simulink library "libaeolus_at"  (Simulink 7.9)
settings: Solver=ode45  StartTime=0.0  StopTime=10.0  RelTol=1e-3
undefined symbols (not defined in the file or in its folder): sigbuilder_block
libraries: simulink x3
(part 2 of 2)

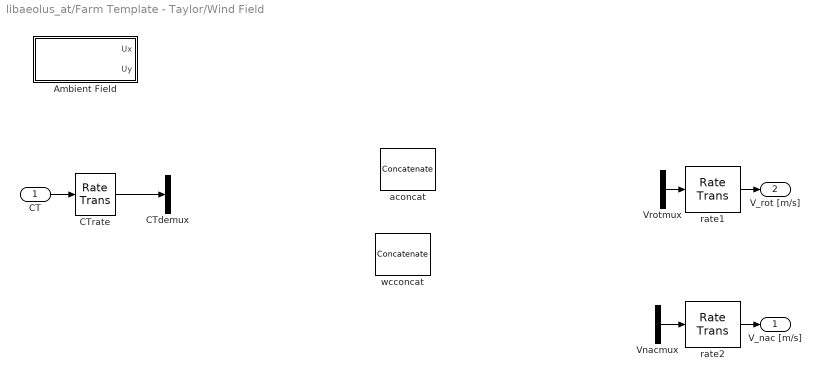
== system libaeolus_at/Farm Template - Taylor/Wind Field ==
  CT : Inport
  Ambient Field : Subsystem
      mask init:
      | wind=get_param(gcb,'UserData');
  CTdemux : Demux  Outputs=3
  CTrate : RateTransition  Deterministic=off  OutPortSampleTime=10
  Vnacmux : Mux  Inputs=2
  Vrotmux : Mux  Inputs=2
  aconcat : Concatenate  Mode=Multidimensional array  ConcatenateDimension=2
  rate1 : RateTransition  Deterministic=off  OutPortSampleTime=SWFTTs
  rate2 : RateTransition  Deterministic=off  OutPortSampleTime=SWFTTs
  wcconcat : Concatenate  Mode=Multidimensional array  ConcatenateDimension=2
  V_nac [m/s] : Outport
  V_rot [m/s] : Outport  Port=2
  wires:
  CT/1 -> CTrate/1
  Vrotmux/1 -> rate1/1
  Vnacmux/1 -> rate2/1
  CTrate/1 -> CTdemux/1
  rate1/1 -> V_rot [m/s]/1
  rate2/1 -> V_nac [m/s]/1

== system libaeolus_at/Farm Template - No Taylor/Network Load/Power Load ==
  Demux : Demux  Tag=STV Demux  Outputs=1
  FromWs : FromWorkspace  Tag=STV FromWs  VariableName=tuvar  SampleTime=0  SigBuilderData=DataTag0  VnvData=DataTag1
      SigBuilderData=|
      | common.afterFinalStr = 'Extrapolate'
      | common.sampleTime = 0
      | dataSet.timeRange = [0 1000]
      | dataSet.name = 'Group 1'
      | sbobj.Groups.Name = 'Group 1'
      | sbobj.Groups.Signals.Name = 'Signal 1'
      | sbobj.Groups.Signals.XData = [0 25 100 200 500 1000]
      | sbobj.Groups.Signals.YData = [0.1 0.1 0.7 0.7 0.9 0.85]
  Signal 1 : Outport  Tag=STV Outport
  wires:
  FromWs/1 -> Demux/1
  Demux/1 -> Signal 1/1

== system libaeolus_at/Farm Template - No Taylor/Post processing/Fatigue Computation ==

== system libaeolus_at/Farm Template - No Taylor/Wind Field/Ambient Lateral Field ==
  Counter Free-Running : simulink/Sources/Counter Free-Running  NumBits=32  tsamp=wind.Ts
  Selector1 : Selector  NumberOfDimensions=2  InputPortWidth=3  IndexOptions=Select all,Index vector (port)  Indices=[1 3],1  OutputSizes=1,1
  Sum : Sum  Inputs=|++
  Turb x : Constant  Value=ceil(wind.grid.xsize/wind.grid.size)-wind.xgrids
  Uy_full : Constant  Value=wind.Uy
  Uy : Outport
  wires:
  Uy_full/1 -> Selector1/1
  Sum/1 -> Selector1/2
  Counter Free-Running/1 -> Sum/2
  Turb x/1 -> Sum/1
  Selector1/1 -> Uy/1

== system libaeolus_at/Farm Template - No Taylor Added Turbulence/Network Load/Power Load ==
  Demux : Demux  Tag=STV Demux  Outputs=1
  FromWs : FromWorkspace  Tag=STV FromWs  VariableName=tuvar  SampleTime=0  SigBuilderData=DataTag2  VnvData=DataTag3
      SigBuilderData=|
      | common.afterFinalStr = 'Extrapolate'
      | common.sampleTime = 0
      | dataSet.timeRange = [0 1000]
      | dataSet.name = 'Group 1'
      | sbobj.Groups.Name = 'Group 1'
      | sbobj.Groups.Signals.Name = 'Signal 1'
      | sbobj.Groups.Signals.XData = [0 25 100 200 500 1000]
      | sbobj.Groups.Signals.YData = [0.1 0.1 0.7 0.7 0.9 0.85]
  Signal 1 : Outport  Tag=STV Outport
  wires:
  Demux/1 -> Signal 1/1
  FromWs/1 -> Demux/1

== system libaeolus_at/Farm Template - No Taylor Added Turbulence/Post processing/Fatigue Computation ==

== system libaeolus_at/Farm Template - No Taylor Added Turbulence/Wind Field/Ambient Lateral Field ==
  Counter Free-Running : simulink/Sources/Counter Free-Running  NumBits=32  tsamp=wind.Ts
  Selector1 : Selector  NumberOfDimensions=2  InputPortWidth=3  IndexOptions=Select all,Index vector (port)  Indices=[1 3],1  OutputSizes=1,1
  Sum : Sum  Inputs=|++
  Turb x : Constant  Value=ceil(wind.grid.xsize/wind.grid.size)-wind.xgrids
  Uy_full : Constant  Value=wind.Uy
  Uy : Outport
  wires:
  Selector1/1 -> Uy/1
  Turb x/1 -> Sum/1
  Counter Free-Running/1 -> Sum/2
  Sum/1 -> Selector1/2
  Uy_full/1 -> Selector1/1

== system libaeolus_at/Farm Template - Taylor/Network Load/Power Load ==
  Demux : Demux  Tag=STV Demux  Outputs=1
  FromWs : FromWorkspace  Tag=STV FromWs  VariableName=tuvar  SampleTime=0  SigBuilderData=DataTag4  VnvData=DataTag5
      SigBuilderData=|
      | common.afterFinalStr = 'Extrapolate'
      | common.sampleTime = 0
      | dataSet.timeRange = [0 1000]
      | dataSet.name = 'Group 1'
      | sbobj.Groups.Name = 'Group 1'
      | sbobj.Groups.Signals.Name = 'Signal 1'
      | sbobj.Groups.Signals.XData = [0 25 100 200 500 1000]
      | sbobj.Groups.Signals.YData = [0.1 0.1 0.7 0.7 0.9 0.85]
  Signal 1 : Outport  Tag=STV Outport
  wires:
  Demux/1 -> Signal 1/1
  FromWs/1 -> Demux/1

== system libaeolus_at/Farm Template - Taylor/Post processing/Fatigue Computation ==

== system libaeolus_at/Farm Template - Taylor/Post processing/Wake Animation ==

== system libaeolus_at/Farm Template - Taylor/Post processing/Wind Field Animation ==

== system libaeolus_at/Farm Template - Taylor/Wind Field/Ambient Field ==
  Counter Free-Running : simulink/Sources/Counter Free-Running  NumBits=32  tsamp=wind.Ts
  Selector : Selector  NumberOfDimensions=2  InputPortWidth=3  IndexOptions=Select all,Index vector (port)  Indices=[1 3],1  OutputSizes=1,1
  Selector1 : Selector  NumberOfDimensions=2  InputPortWidth=3  IndexOptions=Select all,Index vector (port)  Indices=[1 3],1  OutputSizes=1,1
  Sum : Sum  Inputs=|++
  Turb x : Constant  Value=ceil(wind.grid.xsize/wind.grid.size)-wind.xgrids
  Ux_full : Constant  Value=wind.Ux
  Uy_full : Constant  Value=wind.Uy
  Ux : Outport
  Uy : Outport  Port=2
  wires:
  Selector/1 -> Ux/1
  Selector1/1 -> Uy/1
  Turb x/1 -> Sum/1
  Counter Free-Running/1 -> Sum/2
  Sum/1 -> Selector/2, Selector1/2
  Uy_full/1 -> Selector1/1
  Ux_full/1 -> Selector/1

== matlab function Farm Template - No Taylor/Farm Control/control ==
  data: v_nac input double; P_demand input double; parm parameter double; P_ref output double; P_avail output double
function [P_ref,P_avail]  = Farm_Controller(v_nac,P_demand,parm)
%
% Farm_Controller estimates the available power at the farm and distributes the 
% power references proportional to the available power at each wind turbine.
%
% [P_ref,P_avail_total]  = Farm_Controller(v_nac,P_demand)
%
% vn : the wind speed at wind turbine number n.
%
% P_demand : The demanded power by the operator.
%
% P_ref : The power reference for the wind turbines.
%
% P_avail : Available power at the farm level
%
%
% Version 1: 2009-04-10 sms
% Version 2: 2009-12-04 grunnet
% By : S. Mohsen N. Soltani & Jacob D. Grunnet
% Aalborg University, Dept. of Electronic Systems, Section of Automation
% and Control
% E-mail: sms@es.aau.dk
% E-mail: grunnet@es.aau.dk

rho=parm.rho; %air dencity
R=parm.radius; %rotor radius
rated=parm.rated; %Rated power
N=parm.N; %Number of turbines
Cp=parm.Cp; % Max cp of the turbines

P_a=zeros(N,1);
P_ref=zeros(N,1);

% Compute available power at each turbine
for i=1:N
    %P_a=1/2*pi*r^2*Cp*v^3
    P_a(i)=min(rated(i),(pi/2)*rho*R(i)^2*v_nac(i)^3*Cp(i));
end

%Compute total available power
P_avail=sum(P_a);

%Distribute power according to availibility
for i=1:N
    P_ref(i)=max(0,min(rated(i),P_demand*P_a(i)/P_avail));
end

== matlab function Farm Template - No Taylor/Network Operator/Network Operator ==
  data: P_avail input double; settings input double; f input double; P_demand output double; P_demand0 input double; parm parameter double
function P_demand = TSO(P_avail,settings,f,P_demand0,parm)
%
% TSO provides the demanded power to the wind farm controller.
%
% P_avail : Aavailable power at the farm level.
%
% mode : The operation mode.
%
% settings : The settings corresponding to the operational mode
%
% f : Frequency of the network
%
% P_deamnd0 : The last update of the deamded power
%
% Ts : Sample Time
%
% Time-stamp: <2009-04-10 sms>
% Version 1: 2009-04-10 sms 
% By : S. Mohsen N. Soltani
% Aalborg University, Dept. of Electronic Systems, Section of Automation
% and Control
% E-mail: sms@es.aau.dk
% 
 P=0;
 switch(parm.mode)
     case 1 %Absolute active power control
        P=settings(1);
%       % type='Full power';
     case 2 %Delta mode
        P=P_avail-settings(1);
%       % type='Delta mode';
     case 3 %Balance
        P=settings(1);
%       % type='Balance';
     case 4 %Rate limiter
        P=min(P_avail,settings(1)*parm.Ts+P_demand0);
%       % type='Rate limiter';
     case 5 %Frequency Control
        deadb=settings(1);
        contb=settings(2);
        maxp=settings(3);
        minp=settings(4);
        f=f-settings(5); % To provide Delta f
        if ( f<= deadb && f>=-deadb)
            P=0.5*(maxp+minp);
        elseif f>= contb
            P=minp;
        elseif f<= -contb
            P=maxp;
        elseif ( f>deadb && f<contb)
            P=0.5*(maxp+minp)-0.5*(maxp-minp)*(f-deadb)/(contb-deadb);
        elseif ( f<-deadb && f>-contb)
            P=0.5*(maxp+minp)-0.5*(maxp-minp)*(f+deadb)/(contb-deadb);
        end
%       % type='Frequency Control';
     otherwise %Unknown
        P=P_avail;
%       % type='Unknown Mode';
 end
%        

P_demand=max(0,P);

== matlab function Farm Template - No Taylor/Wind Field/Deficit ==
  data: w_c input double; w_d input double; ct_dw input double; p parameter double; def output double; turb output double
function [def, turb] = deficit(w_c,w_d,ct_dw,p) %#eml
% w_c   is the vector of wake centers from the other turbins at the x position of the turbine
% w_d   is the vector of wake diameters from the other turbins at the x position of the turbine
% ct_dw is the vector of thrust coefficients from the other turbins at the x position of the turbine
% p     is a structure containing farm layout and tubine rotor sizes  

wake_from = zeros(length(p.farm.x),length(p.farm.x));
dist_i = zeros(length(p.farm.x),1);
def = ones(length(p.farm.x),1);
turb = ones(length(p.farm.x),1);

if ct_dw(size(ct_dw,1),1) ~= 0 % only calculate deficit if wind has reached end of farm
    [~, dist_i] = sort(p.farm.x);

    %This for-loop make a "tree" of which turbines are in the wake
    for i=1:length(p.farm.x)
        turb_i = dist_i(i);
        for k = 1:length(p.farm.x)
            turb_k = dist_i(k);
            temp = p.farm.y(turb_k)-w_c(turb_k,turb_i);
            %if turb_k is in turb_i's wake it is included in the "tree"
            if(temp > -w_d(turb_k,turb_i) && temp < w_d(turb_k,turb_i))  
                wake_from(i,k) = 1; %
            end
        end
    end
    wake_from_2 = wake_from; %copy original wake tree for later use

    for i=1:length(p.farm.x)
        % remove parents from tree if children is in wake = use iterative scheme
        pp = find(wake_from(:,i)==1);
        c = find(wake_from(i,:)==1);
        wake_from(pp,c) = 0;
        switch length(pp)
            case 0 % if no wake the deficit is one    %similar for 'turbulence gain'
                def(i) = 1;
                turb(i) = 1;
            case 1 % if one wake then calculate deficit using iterative scheme
                wake_upstream = find(wake_from_2(:,i)==1); %find the upstream turbines
                wd = w_d(dist_i(i),dist_i(min(wake_upstream))); %find wake diameter for "most" upstream turbine
                tmp_ct = ct_dw(dist_i(i),dist_i(max(wake_upstream))); % find CT for closest upstream turbine
                tmp_rotor_D = 2*p.rotor.r(dist_i(max(wake_upstream))); % precalculate rotor diameter for closest upstream turbine
                if(length(wake_upstream) == 1) % if only one upstream turbine use "normal" deficit calculation
                    def(i) = 1-0.5*tmp_rotor_D^2/wd^2*tmp_ct;
                else % else use iterative scheme : "Analytical Modelling of Wind Speed Deficit in Large Offshore Wind Farms" eq:17
                    tmp_def = def(max(wake_upstream)); %find deficit at closest upstream turbine
                    tmp_D = w_d(dist_i(max(wake_upstream)),dist_i(min(wake_upstream))); %find diameter of wake at closest upstream turbine
                    def(i) = 1-(tmp_D^2/wd^2*(1-tmp_def)+0.5*tmp_rotor_D^2/wd^2*tmp_ct*tmp_def); %calculate deficit
                end
            otherwise % if more than wakes meet (overlap but not in row) merge according to area
                %error = 1 % uncomment to see when wakes are merged from other rows
                wake_upstream = find(wake_from_2(:,i)==1);
                wd = w_d(dist_i(i),dist_i(min(wake_upstream)));
                tmp_def = ones(length(pp),1);
                tmp_D = ones(length(pp),1);
                k = 1;
                for l=length(pp) %calculate deficit from each upstream turbine
                    j = pp(l);
                    tmp_ct = ct_dw(dist_i(i),dist_i(j));
                    tmp_def_up = def(dist_i(j));
                    tmp_rotor_D = 2*p.rotor.r(dist_i(max(wake_upstream)));
                    tmp_D(k) = w_d(dist_i(j),dist_i(min(wake_upstream)));
                    tmp_def(k) = 1-(tmp_D(k)^2/wd^2*(1-tmp_def_up)+0.5*tmp_rotor_D^2/wd^2*tmp_ct*tmp_def_up);
                    k = k+1;
                end
                def(i) = sum(tmp_D.^2.*tmp_def)/sum(tmp_D.^2); %combine deficit according to area
        end
    end
    def(dist_i) = def; % Reshuffle deficits such that turbine number is correct
end

== matlab function Farm Template - No Taylor Added Turbulence/Farm Control/control ==
  data: v_nac input double; P_demand input double; parm parameter double; P_ref output double; P_avail output double
function [P_ref,P_avail]  = Farm_Controller(v_nac,P_demand,parm)
%
% Farm_Controller estimates the available power at the farm and distributes the 
% power references proportional to the available power at each wind turbine.
%
% [P_ref,P_avail_total]  = Farm_Controller(v_nac,P_demand)
%
% vn : the wind speed at wind turbine number n.
%
% P_demand : The demanded power by the operator.
%
% P_ref : The power reference for the wind turbines.
%
% P_avail : Available power at the farm level
%
%
% Version 1: 2009-04-10 sms
% Version 2: 2009-12-04 grunnet
% By : S. Mohsen N. Soltani & Jacob D. Grunnet
% Aalborg University, Dept. of Electronic Systems, Section of Automation
% and Control
% E-mail: sms@es.aau.dk
% E-mail: grunnet@es.aau.dk

rho=parm.rho; %air dencity
R=parm.radius; %rotor radius
rated=parm.rated; %Rated power
N=parm.N; %Number of turbines
Cp=parm.Cp; % Max cp of the turbines

P_a=zeros(N,1);
P_ref=zeros(N,1);

% Compute available power at each turbine
for i=1:N
    %P_a=1/2*pi*r^2*Cp*v^3
    P_a(i)=min(rated(i),(pi/2)*rho*R(i)^2*v_nac(i)^3*Cp(i));
end

%Compute total available power
P_avail=sum(P_a);

%Distribute power according to availibility
for i=1:N
    P_ref(i)=max(0,min(rated(i),P_demand*P_a(i)/P_avail));
end

== matlab function Farm Template - No Taylor Added Turbulence/Network Operator/Network Operator ==
  data: P_avail input double; settings input double; f input double; P_demand output double; P_demand0 input double; parm parameter double
function P_demand = TSO(P_avail,settings,f,P_demand0,parm)
%
% TSO provides the demanded power to the wind farm controller.
%
% P_avail : Aavailable power at the farm level.
%
% mode : The operation mode.
%
% settings : The settings corresponding to the operational mode
%
% f : Frequency of the network
%
% P_deamnd0 : The last update of the deamded power
%
% Ts : Sample Time
%
% Time-stamp: <2009-04-10 sms>
% Version 1: 2009-04-10 sms 
% By : S. Mohsen N. Soltani
% Aalborg University, Dept. of Electronic Systems, Section of Automation
% and Control
% E-mail: sms@es.aau.dk
% 
 P=0;
 switch(parm.mode)
     case 1 %Absolute active power control
        P=settings(1);
%       % type='Full power';
     case 2 %Delta mode
        P=P_avail-settings(1);
%       % type='Delta mode';
     case 3 %Balance
        P=settings(1);
%       % type='Balance';
     case 4 %Rate limiter
        P=min(P_avail,settings(1)*parm.Ts+P_demand0);
%       % type='Rate limiter';
     case 5 %Frequency Control
        deadb=settings(1);
        contb=settings(2);
        maxp=settings(3);
        minp=settings(4);
        f=f-settings(5); % To provide Delta f
        if ( f<= deadb && f>=-deadb)
            P=0.5*(maxp+minp);
        elseif f>= contb
            P=minp;
        elseif f<= -contb
            P=maxp;
        elseif ( f>deadb && f<contb)
            P=0.5*(maxp+minp)-0.5*(maxp-minp)*(f-deadb)/(contb-deadb);
        elseif ( f<-deadb && f>-contb)
            P=0.5*(maxp+minp)-0.5*(maxp-minp)*(f+deadb)/(contb-deadb);
        end
%       % type='Frequency Control';
     otherwise %Unknown
        P=P_avail;
%       % type='Unknown Mode';
 end
%        

P_demand=max(0,P);

== matlab function Farm Template - No Taylor Added Turbulence/Wind Field/Deficit and turbulence ==
  data: w_c input double; w_d input double; ct_dw input double; p parameter double; def output double; turb output double
function [def, turb] = deficit(w_c,w_d,ct_dw,p) %#eml
% w_c   is the vector of wake centers from the other turbins at the x position of the turbine
% w_d   is the vector of wake diameters from the other turbins at the x position of the turbine
% ct_dw is the vector of thrust coefficients from the other turbins at the x position of the turbine
% p     is a structure containing farm layout and tubine rotor sizes  

wake_from = zeros(length(p.farm.x),length(p.farm.x));
dist_i = zeros(length(p.farm.x),1);
def = ones(length(p.farm.x),1);

turb = ones(length(p.farm.x),1);
sigma0 = p.sigma0; %ambient wind speed turbulence intensity
U0 = p.U0; %ambient wind speed mean 

if ct_dw(size(ct_dw,1),1) ~= 0 % only calculate deficit if wind has reached end of farm
    [~, dist_i] = sort(p.farm.x);

    %This for-loop make a "tree" of which turbines are in the wake
    for i=1:length(p.farm.x)
        turb_i = dist_i(i);
        for k = 1:length(p.farm.x)
            turb_k = dist_i(k);
            temp = p.farm.y(turb_k)-w_c(turb_k,turb_i);
            %if turb_k is in turb_i's wake it is included in the "tree"
            if(temp > -w_d(turb_k,turb_i) && temp < w_d(turb_k,turb_i))  
                wake_from(i,k) = 1; %
            end
        end
    end
    wake_from_2 = wake_from; %copy original wake tree for later use

    for i=1:length(p.farm.x)
        % remove parents from tree if children is in wake = use iterative scheme
        pp = find(wake_from(:,i)==1);
        c = find(wake_from(i,:)==1);
        wake_from(pp,c) = 0;
        switch length(pp)
            case 0 % if no wake the deficit/turbulence is one
                def(i) = 1;
                turb(i) = 1;
            case 1 % if one wake then calculate deficit using iterative scheme
                wake_upstream = find(wake_from_2(:,i)==1); %find the upstream turbines
                wd = w_d(dist_i(i),dist_i(min(wake_upstream))); %find wake diameter for "most" upstream turbine
                tmp_ct = ct_dw(dist_i(i),dist_i(max(wake_upstream))); % find CT for closest upstream turbine
                tmp_rotor_D = 2*p.rotor.r(dist_i(max(wake_upstream))); % precalculate rotor diameter for closest upstream turbine
                if(length(wake_upstream) == 1) % if only one upstream turbine use "normal" deficit calculation
                    def(i) = 1-0.5*tmp_rotor_D^2/wd^2*tmp_ct;
                else % else use iterative scheme : "Analytical Modelling of Wind Speed Deficit in Large Offshore Wind Farms" eq:17
                    tmp_def = def(max(wake_upstream)); %find deficit at closest upstream turbine
                    tmp_D = w_d(dist_i(max(wake_upstream)),dist_i(min(wake_upstream))); %find diameter of wake at closest upstream turbine
                    def(i) = 1-(tmp_D^2/wd^2*(1-tmp_def)+0.5*tmp_rotor_D^2/wd^2*tmp_ct*tmp_def); %calculate deficit
                end
                    
                %Euclidean distance Edist between turbine in wake and closest wake generating turbine
                Edist = sqrt((p.farm.x(dist_i(i)) - p.farm.x(dist_i(max(wake_upstream))))^2 + ...
                (p.farm.y(dist_i(i)) - p.farm.y(dist_i(max(wake_upstream))))^2);
                %added turbulence sigma_add, eq (4.14) in Frandsen thesis
                sigma_add = (U0*def(i))/(1.5 + 0.8*((Edist/tmp_rotor_D)/sqrt(abs(tmp_ct)))); 
                %added turbulence scaling parameter turb, rearranged from
                %eq (3.17) in Frandsen such that sigma_Turbine = turb*sigma0
                turb(i) = sqrt((sigma_add/(sigma0*U0))^2 + 1); %we multiply with U0 in denominator since sigma0 is actually ambient turbulence intensity
            otherwise % if more than wakes meet (overlap but not in row) merge according to area
                %error = 1 % uncomment to see when wakes are merged from other rows
                wake_upstream = find(wake_from_2(:,i)==1);
                wd = w_d(dist_i(i),dist_i(min(wake_upstream)));
                tmp_def = ones(length(pp),1);
                tmp_D = ones(length(pp),1);
                
                tmp_turb = ones(length(pp),1);
                k = 1;
                for l=length(pp) %calculate deficit from each upstream turbine
                    j = pp(l);
                    tmp_ct = ct_dw(dist_i(i),dist_i(j));
                    tmp_def_up = def(dist_i(j));
                    tmp_rotor_D = 2*p.rotor.r(dist_i(max(wake_upstream)));
                    tmp_D(k) = w_d(dist_i(j),dist_i(min(wake_upstream)));
                    tmp_def(k) = 1-(tmp_D(k)^2/wd^2*(1-tmp_def_up)+0.5*tmp_rotor_D^2/wd^2*tmp_ct*tmp_def_up);
 
                    k = k+1;
                end
                def(i) = sum(tmp_D.^2.*tmp_def)/sum(tmp_D.^2); %combine deficit according to area
                k = 1;
                for l=length(pp) %calculate deficit from each upstream turbine
                    j = pp(l);
                    tmp_ct = ct_dw(dist_i(i),dist_i(j));
                    
                    Edist = sqrt((p.farm.x(dist_i(i)) - p.farm.x(dist_i(j)))^2 + ...
                    (p.farm.y(dist_i(i)) - p.farm.y(dist_i(j)))^2);%should dist_i(j) be dist_i(max(wake_upstream)) here?
                    tmp_rotor_D_turb = 2*p.rotor.r(dist_i(j));
                    sigma_add = (U0*def(i))/(1.5 + 0.8*((Edist/tmp_rotor_D_turb)/sqrt(abs(tmp_ct))));
                    tmp_turb(k) = sqrt((sigma_add/(sigma0*U0))^2 + 1); %we multiply with U0 in denominator since sigma0 is actually ambient turbulence intensity
                    k = k+1;
                end
                turb(i) = sum(tmp_D.^2.*tmp_turb)/sum(tmp_D.^2); %combine turbulence according to area
        end
    end
    def(dist_i) = def; % Reshuffle deficits/turbulence such that turbine number is correct
    turb(dist_i) = turb;
end

== matlab function Farm Template - Taylor/Farm Control/control ==
  data: v_nac input double; P_demand input double; parm parameter double; P_ref output double; P_avail output double
function [P_ref,P_avail]  = Farm_Controller(v_nac,P_demand,parm)
%
% Farm_Controller estimates the available power at the farm and distributes the 
% power references proportional to the available power at each wind turbine.
%
% [P_ref,P_avail_total]  = Farm_Controller(v_nac,P_demand)
%
% vn : the wind speed at wind turbine number n.
%
% P_demand : The demanded power by the operator.
%
% P_ref : The power reference for the wind turbines.
%
% P_avail : Available power at the farm level
%
%
% Version 1: 2009-04-10 sms
% Version 2: 2009-12-04 grunnet
% By : S. Mohsen N. Soltani & Jacob D. Grunnet
% Aalborg University, Dept. of Electronic Systems, Section of Automation
% and Control
% E-mail: sms@es.aau.dk
% E-mail: grunnet@es.aau.dk

rho=parm.rho; %air dencity
R=parm.radius; %rotor radius
rated=parm.rated; %Rated power
N=parm.N; %Number of turbines
Cp=parm.Cp; % Max cp of the turbines

P_a=zeros(N,1);
P_ref=zeros(N,1);

% Compute available power at each turbine
for i=1:N
    %P_a=1/2*pi*r^2*Cp*v^3
    P_a(i)=min(rated(i),(pi/2)*rho*R(i)^2*v_nac(i)^3*Cp(i));
end

%Compute total available power
P_avail=sum(P_a);

%Distribute power according to availibility
for i=1:N
    P_ref(i)=max(0,min(rated(i),P_demand*P_a(i)/P_avail));
end

== matlab function Farm Template - Taylor/Network Operator/Network Operator ==
  data: P_avail input double; settings input double; f input double; P_demand output double; P_demand0 input double; parm parameter double
function P_demand = TSO(P_avail,settings,f,P_demand0,parm)
%
% TSO provides the demanded power to the wind farm controller.
%
% P_avail : Aavailable power at the farm level.
%
% mode : The operation mode.
%
% settings : The settings corresponding to the operational mode
%
% f : Frequency of the network
%
% P_deamnd0 : The last update of the deamded power
%
% Ts : Sample Time
%
% Time-stamp: <2009-04-10 sms>
% Version 1: 2009-04-10 sms 
% By : S. Mohsen N. Soltani
% Aalborg University, Dept. of Electronic Systems, Section of Automation
% and Control
% E-mail: sms@es.aau.dk
% 
 P=0;
 switch(parm.mode)
     case 1 %Absolute active power control
        P=settings(1);
%       % type='Full power';
     case 2 %Delta mode
        P=P_avail-settings(1);
%       % type='Delta mode';
     case 3 %Balance
        P=settings(1);
%       % type='Balance';
     case 4 %Rate limiter
        P=min(P_avail,settings(1)*parm.Ts+P_demand0);
%       % type='Rate limiter';
     case 5 %Frequency Control
        deadb=settings(1);
        contb=settings(2);
        maxp=settings(3);
        minp=settings(4);
        f=f-settings(5); % To provide Delta f
        if ( f<= deadb && f>=-deadb)
            P=0.5*(maxp+minp);
        elseif f>= contb
            P=minp;
        elseif f<= -contb
            P=maxp;
        elseif ( f>deadb && f<contb)
            P=0.5*(maxp+minp)-0.5*(maxp-minp)*(f-deadb)/(contb-deadb);
        elseif ( f<-deadb && f>-contb)
            P=0.5*(maxp+minp)-0.5*(maxp-minp)*(f+deadb)/(contb-deadb);
        end
%       % type='Frequency Control';
     otherwise %Unknown
        P=P_avail;
%       % type='Unknown Mode';
 end
%        

P_demand=max(0,P);
